simulink model "BMS"  (R2021a)
settings: Solver=FixedStepDiscrete  StartTime=0.0  StopTime=inf  FixedStep=1  RelTol=1e-3
values from neighbouring files (symbols this model uses):
  BattTempBp = [243.1 253.1 263.1 273.1 283.1 298.1 313.1]*0.1    [Variables.m]
  BM_TiCtctrCnct_P = single(1)/BMS_TiSample_C    [Variables.m]
  BM_TiCtctrDCnct_P = single(1)/BMS_TiSample_C    [Variables.m]
  BMS_EnaFltSts = [1 1 1 1 1 1 1 1 0 0 0 0 0]    [Variables.m]
  BMS_ModeEnaFltChk = [0 100 110 111 115 120 130 140 200 211 220 230 255]    [Variables.m]
  BMS_TiSample_C = single(0.1)    [Variables.m]
  BPC_BattTotalCharge_P = single(48)    [Variables.m]
  BPC_BattTotalEnergy_P = BPC_BattTotalCharge_P * single(NrCells_C) * CVM_VCellMaxCutoffTh_P    [Variables.m]
  CapLUTBp = [0 0.01 0.02 0.03 0.04 0.05 0.06 0.07 0.08 0.09 0.1 0.11 0.12 0.13 0.14 0.15 0.16 0.17 0.18 0.19 0.2 0.21 0.22 0.23 0.24 0.25 0.26 0.27 0.28 0.29 0.3 0.31 0.32 0.33 0.34 0.35 0.36 0.37 0.38 0.39 0.4 0.41 0.42 0.43 0.44 0.45 0.46 0.47 0.48 0.49 0.5 0.51 0.52 0.53 0.54 0.55 0.56 0.57 0.58 0.59 0.6 0.61 0.62 0.63 0.64 0.65 0.66 0.67 0.68 0.69 0.7 0.71 0.72 0.73 0.74 0.75 0.76 0.77 0.78 0.79 0.8 0.81  ...(+91 chars)    [Variables.m]
  CapSOCBp = [0 0.2 0.4 0.6 0.8 1]    [Variables.m]
  CVM_DMaxVCellMaxCutoff_P = int16(0.5/BMS_TiSample_C)    [Variables.m]
  CVM_DMaxVCellMaxDrtd_P = int16(0.5/BMS_TiSample_C)    [Variables.m]
  CVM_DMaxVCellMaxWarn_P = int16(0.5/BMS_TiSample_C)    [Variables.m]
  CVM_DMaxVCellMinCutoff_P = int16(0.5/BMS_TiSample_C)    [Variables.m]
  CVM_DMaxVCellMinDrtd_P = int16(0.5/BMS_TiSample_C)    [Variables.m]
  CVM_DMaxVCellMinWarn_P = int16(0.5/BMS_TiSample_C)    [Variables.m]
  CVM_DMinVCellMaxCutoff_P = -int16(0.5/BMS_TiSample_C)    [Variables.m]
  CVM_DMinVCellMaxDrtd_P = -int16(0.5/BMS_TiSample_C)    [Variables.m]
  CVM_DMinVCellMaxWarn_P = -int16(0.5/BMS_TiSample_C)    [Variables.m]
  CVM_DMinVCellMinCutoff_P = -int16(0.5/BMS_TiSample_C)    [Variables.m]
  CVM_DMinVCellMinDrtd_P = -int16(0.5/BMS_TiSample_C)    [Variables.m]
  CVM_DMinVCellMinWarn_P = -int16(0.5/BMS_TiSample_C)    [Variables.m]
  CVM_VCellMaxCutoffTh_P = single(4.22)    [Variables.m]
  CVM_VCellMaxDrtdTh_P = single(4.15)    [Variables.m]
  CVM_VCellMaxWarnTh_P = single(4.1)    [Variables.m]
  CVM_VCellMinCutoffTh_P = single(3.26)    [Variables.m]
  CVM_VCellMinDrtdTh_P = single(3)    [Variables.m]
  CVM_VCellMinWarnTh_P = single(2.8)    [Variables.m]
  Em = [2.8 3.228 3.284 3.361 3.408 3.427 3.472 3.477 3.493 3.504 3.516 3.528 3.537 3.545 3.555 3.561 3.566 3.576 3.587 3.589 3.594 3.6 3.608 3.61 3.616 3.619 3.626 3.632 3.637 3.64 3.645 3.646 3.652 3.655 3.658 3.661 3.664 3.668 3.673 3.678 3.68 3.681 3.686 3.692 3.699 3.702 3.705 3.71 3.717 3.723 3.728 3.733 3.735 3.742 3.749 3.755 3.761 3.768 3.773 3.78 3.791 3.798 3.798 3.814 3.818 3.825 3.841 3.846  ...(+196 chars)    [Variables.m]
  MTM_DMaxTMdulMaxCutoff_P = int16(0.5/BMS_TiSample_C)    [Variables.m]
  MTM_DMaxTMdulMaxDrtd_P = int16(0.5/BMS_TiSample_C)    [Variables.m]
  MTM_DMaxTMdulMaxWarn_P = int16(0.5/BMS_TiSample_C)    [Variables.m]
  MTM_DMaxTMdulMinCutoff_P = int16(0.5/BMS_TiSample_C)    [Variables.m]
  MTM_DMaxTMdulMinDrtd_P = int16(0.5/BMS_TiSample_C)    [Variables.m]
  MTM_DMaxTMdulMinWarn_P = int16(0.5/BMS_TiSample_C)    [Variables.m]
  MTM_DMinTMdulMaxCutoff_P = -int16(0.5/BMS_TiSample_C)    [Variables.m]
  MTM_DMinTMdulMaxDrtd_P = -int16(0.5/BMS_TiSample_C)    [Variables.m]
  MTM_DMinTMdulMaxWarn_P = -int16(0.5/BMS_TiSample_C)    [Variables.m]
  MTM_DMinTMdulMinCutoff_P = -int16(0.5/BMS_TiSample_C)    [Variables.m]
  MTM_DMinTMdulMinDrtd_P = -int16(0.5/BMS_TiSample_C)    [Variables.m]
  MTM_DMinTMdulMinWarn_P = -int16(0.5/BMS_TiSample_C)    [Variables.m]
  MTM_TMdulMaxCutoffTh_P = single(55)    [Variables.m]
  MTM_TMdulMaxDrtdTh_P = single(52.5)    [Variables.m]
  MTM_TMdulMaxWarnTh_P = single(50)    [Variables.m]
  MTM_TMdulMinCutoffTh_P = single(-20)    [Variables.m]
  MTM_TMdulMinDrtdTh_P = single(0)    [Variables.m]
  MTM_TMdulMinWarnTh_P = single(5)    [Variables.m]
  NrCutoff_C = uint8(3)    [Variables.m]
  NrDrtd_C = uint8(2)    [Variables.m]
  NrNoFlt_C = uint8(0)    [Variables.m]
  NrTMdulSnsr_C = uint8(3)    [Variables.m]
  NrWarn_C = uint8(1)    [Variables.m]
  RInt = [0.008846 0.009319 0.009027 0.00847 0.01032 0.01314;0.006389 0.006554 0.005553 0.005525 0.006043 0.007805;0.004364 0.004101 0.00406 0.003452 0.003846 0.004517;0.002031 0.002563 0.002532 0.00246 0.002716 0.003047;0.001443 0.001825 0.001795 0.001778 0.001924 0.002234;0.0005603 0.0007192 0.0006887 0.0007557 0.0007355 0.001014;0.001028 0.001338 0.001 0.001536 0.001546 0.002789]    [Variables.m]
undefined symbols (not defined in the file or in its folder): DiscIntNeverNeededParam
libraries: BMSLib x12
settings Model: Creator=Santosh  LastModifiedBy=Kuhan
settings SolverCC: AlgebraicLoopSolver=TrustRegion
settings DataIOCC: ReturnWorkspaceOutputs=off
settings DebuggingCC: SFMachineParentedDataDiag=warning  ArithmeticOperatorsInVariantConditions=warning
settings SFSimCC: CustomCodeUndefinedFunction=UseInterfaceOnly

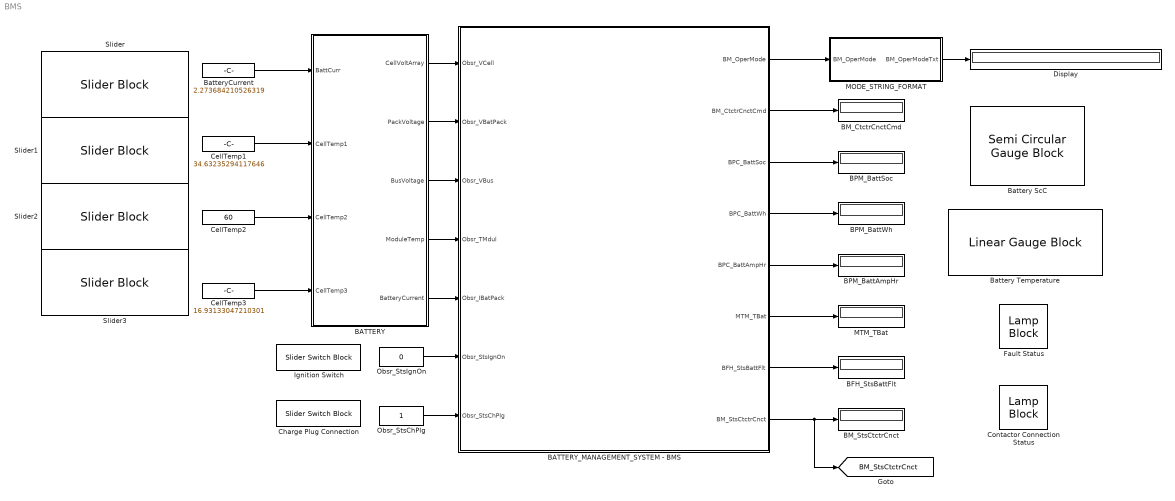
== system BMS ==
  BATTERY : Subsystem
  BATTERY_MANAGEMENT_SYSTEM - BMS : Subsystem
  BFH_StsBattFlt : Display
  BM_CtctrCnctCmd : Display
  BM_StsCtctrCnct : Display
  BPM_BattAmpHr : Display
  BPM_BattSoc : Display
  BPM_BattWh : Display
  Battery ScC : SemiCircularGaugeBlock
  Battery Temperature : LinearGaugeBlock  ScaleMin=-60  ScaleMax=60
  BatteryCurrent : Constant  Value=2.273684210526319  OutDataTypeStr=double
  CellTemp1 : Constant  Value=34.63235294117646  OutDataTypeStr=double
  CellTemp2 : Constant  Value=60  OutDataTypeStr=double
  CellTemp3 : Constant  Value=16.93133047210301  OutDataTypeStr=double
  Charge Plug Connection : SliderSwitchBlock
      settings: Values={{'Off', 'On'}, [0 1]}
  Contactor Connection Status : LampBlock
  Display : Display
  Fault Status : LampBlock
  Ignition Switch : SliderSwitchBlock
      settings: Values={{'Off', 'On'}, [0 1]}
  MODE_STRING_FORMAT : Subsystem
  MTM_TBat : Display
  Obsr_StsChPlg : Constant  OutDataTypeStr=boolean
  Obsr_StsIgnOn : Constant  Value=0  OutDataTypeStr=boolean
  Slider : SliderBlock  ScaleMin=-24  ScaleMax=24
  Slider1 : SliderBlock  ScaleMin=-30  ScaleMax=60
  Slider2 : SliderBlock  ScaleMin=-30  ScaleMax=60
  Slider3 : SliderBlock  ScaleMin=-30  ScaleMax=60
  tag scope: BM_StsCtctrCnct=global
  wires:
  Obsr_StsIgnOn/1 -> BATTERY_MANAGEMENT_SYSTEM - BMS/6(Obsr_StsIgnOn)
  Obsr_StsChPlg/1 -> BATTERY_MANAGEMENT_SYSTEM - BMS/7(Obsr_StsChPlg)
  BATTERY_MANAGEMENT_SYSTEM - BMS/3(BPC_BattSoc) -> BPM_BattSoc/1
  BATTERY_MANAGEMENT_SYSTEM - BMS/2(BM_CtctrCnctCmd) -> BM_CtctrCnctCmd/1
  BATTERY_MANAGEMENT_SYSTEM - BMS/4(BPC_BattWh) -> BPM_BattWh/1
  BATTERY_MANAGEMENT_SYSTEM - BMS/5(BPC_BattAmpHr) -> BPM_BattAmpHr/1
  BATTERY_MANAGEMENT_SYSTEM - BMS/6(MTM_TBat) -> MTM_TBat/1
  BATTERY_MANAGEMENT_SYSTEM - BMS/7(BFH_StsBattFlt) -> BFH_StsBattFlt/1
  BATTERY_MANAGEMENT_SYSTEM - BMS/8(BM_StsCtctrCnct) -> BM_StsCtctrCnct/1, [BM_StsCtctrCnct]
  BATTERY/1(CellVoltArray) -> BATTERY_MANAGEMENT_SYSTEM - BMS/1(Obsr_VCell)
  BATTERY/2(PackVoltage) -> BATTERY_MANAGEMENT_SYSTEM - BMS/2(Obsr_VBatPack)
  BATTERY/3(BusVoltage) -> BATTERY_MANAGEMENT_SYSTEM - BMS/3(Obsr_VBus)
  BATTERY/4(ModuleTemp) -> BATTERY_MANAGEMENT_SYSTEM - BMS/4(Obsr_TMdul)
  BATTERY/5(BatteryCurrent) -> BATTERY_MANAGEMENT_SYSTEM - BMS/5(Obsr_IBatPack)
  CellTemp1/1 -> BATTERY/2(CellTemp1)
  CellTemp2/1 -> BATTERY/3(CellTemp2)
  CellTemp3/1 -> BATTERY/4(CellTemp3)
  BATTERY_MANAGEMENT_SYSTEM - BMS/1(BM_OperMode) -> MODE_STRING_FORMAT/1(BM_OperMode)
  BatteryCurrent/1 -> BATTERY/1(BattCurr)
  MODE_STRING_FORMAT/1(BM_OperModeTxt) -> Display/1

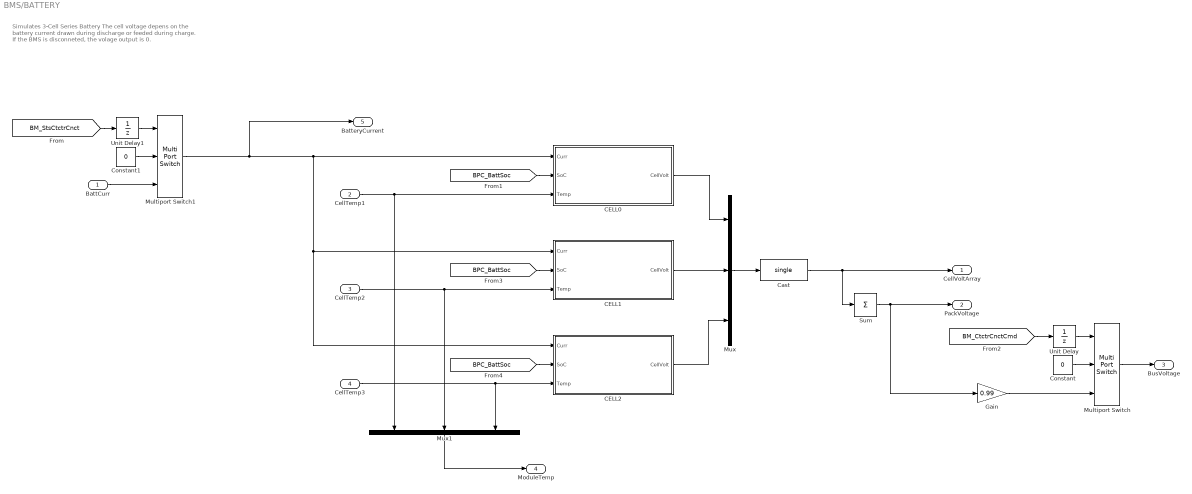
== system BMS/BATTERY ==
  note: Simulates 3-Cell Series Battery
      |
      | The cell voltage depens on the battery current drawn during discharge or feeded during charge.
      |
      | If the BMS is disconneted, the volage output is 0.
  BattCurr : Inport
  CellTemp1 : Inport  Port=2
  CellTemp2 : Inport  Port=3
  CellTemp3 : Inport  Port=4
  CELL0 : Subsystem
  CELL1 : Subsystem
  CELL2 : Subsystem
  Cast : DataTypeConversion  OutDataTypeStr=single
  Constant : Constant  Value=0
  Constant1 : Constant  Value=0
  Gain : Gain  Gain=0.99  OutDataTypeStr=single
  Multiport Switch : MultiPortSwitch  DataPortOrder=Zero-based contiguous  Inputs=2  zeroidx=on  OutDataTypeStr=single
  Multiport Switch1 : MultiPortSwitch  DataPortOrder=Zero-based contiguous  Inputs=2  zeroidx=on
  Mux : Mux  Inputs=3
  Mux1 : Mux  Inputs=3
  Sum : Sum  Inputs=1  AccumDataTypeStr=single
  Unit Delay : UnitDelay  SampleTime=-1  HasFrameUpgradeWarning=on
  Unit Delay1 : UnitDelay  SampleTime=-1  HasFrameUpgradeWarning=on
  CellVoltArray : Outport  VectorParamsAs1DForOutWhenUnconnected=off
  PackVoltage : Outport  Port=2  VectorParamsAs1DForOutWhenUnconnected=off
  BusVoltage : Outport  Port=3  VectorParamsAs1DForOutWhenUnconnected=off
  ModuleTemp : Outport  Port=4  VectorParamsAs1DForOutWhenUnconnected=off
  BatteryCurrent : Outport  Port=5  VectorParamsAs1DForOutWhenUnconnected=off
  wires:
  CellTemp2/1 -> CELL1/3(Temp), Mux1/2
  CELL1/1(CellVolt) -> Mux/2
  CellTemp3/1 -> CELL2/3(Temp), Mux1/3
  CELL2/1(CellVolt) -> Mux/3
  CELL0/1(CellVolt) -> Mux/1
  CellTemp1/1 -> CELL0/3(Temp), Mux1/1
  Mux/1 -> Cast/1
  Sum/1 -> PackVoltage/1, Gain/1
  Mux1/1 -> ModuleTemp/1
  Cast/1 -> Sum/1, CellVoltArray/1
  Multiport Switch1/1 -> CELL0/1(Curr), CELL2/1(Curr), CELL1/1(Curr), BatteryCurrent/1
  Unit Delay/1 -> Multiport Switch/1
  [BM_CtctrCnctCmd] -> Unit Delay/1
  Multiport Switch/1 -> BusVoltage/1
  Gain/1 -> Multiport Switch/3
  Constant/1 -> Multiport Switch/2
  Unit Delay1/1 -> Multiport Switch1/1
  [BM_StsCtctrCnct] -> Unit Delay1/1
  Constant1/1 -> Multiport Switch1/2
  BattCurr/1 -> Multiport Switch1/3
  [BPC_BattSoc] -> CELL0/2(SoC)
  [BPC_BattSoc] -> CELL1/2(SoC)
  [BPC_BattSoc] -> CELL2/2(SoC)

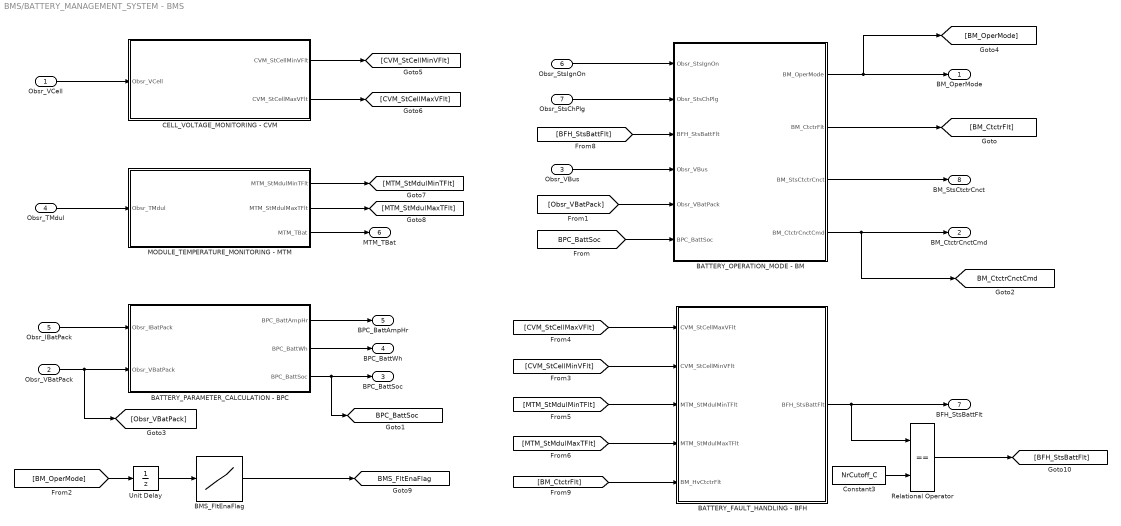
== system BMS/BATTERY_MANAGEMENT_SYSTEM - BMS ==
  Obsr_VCell : Inport
  Obsr_VBatPack : Inport  Port=2
  Obsr_VBus : Inport  Port=3
  Obsr_TMdul : Inport  Port=4
  Obsr_IBatPack : Inport  Port=5
  Obsr_StsIgnOn : Inport  Port=6
  Obsr_StsChPlg : Inport  Port=7
  BATTERY_FAULT_HANDLING - BFH : Subsystem
  BATTERY_OPERATION_MODE - BM : Subsystem
  BATTERY_PARAMETER_CALCULATION - BPC : Subsystem
  BMS_FltEnaFlag : Lookup_n-D  NumberOfTableDimensions=1  BreakpointsForDimension1=BMS_ModeEnaFltChk  Table=BMS_EnaFltSts  InterpMethod=Nearest  ExtrapMethod=Clip  DiagnosticForOutOfRangeInput=Error  InternalRulePriority=Speed  RndMeth=Simplest  InputSameDT=on
  CELL_VOLTAGE_MONITORING - CVM : Subsystem
  Constant3 : Constant  Value=NrCutoff_C
  MODULE_TEMPERATURE_MONITORING - MTM : Subsystem
  Relational Operator : RelationalOperator  Operator===  OutDataTypeStr=boolean  RndMeth=Simplest
  Unit Delay : UnitDelay  SampleTime=-1  HasFrameUpgradeWarning=on
  BM_OperMode : Outport  VectorParamsAs1DForOutWhenUnconnected=off
  BM_CtctrCnctCmd : Outport  Port=2  VectorParamsAs1DForOutWhenUnconnected=off
  BPC_BattSoc : Outport  Port=3  VectorParamsAs1DForOutWhenUnconnected=off
  BPC_BattWh : Outport  Port=4  VectorParamsAs1DForOutWhenUnconnected=off
  BPC_BattAmpHr : Outport  Port=5  VectorParamsAs1DForOutWhenUnconnected=off
  MTM_TBat : Outport  Port=6  VectorParamsAs1DForOutWhenUnconnected=off
  BFH_StsBattFlt : Outport  Port=7  VectorParamsAs1DForOutWhenUnconnected=off
  BM_StsCtctrCnct : Outport  Port=8  VectorParamsAs1DForOutWhenUnconnected=off
  tag scope: BMS_FltEnaFlag=global, BM_CtctrCnctCmd=global, BPC_BattSoc=global
  wires:
  Obsr_VCell/1 -> CELL_VOLTAGE_MONITORING - CVM/1(Obsr_VCell)
  Obsr_TMdul/1 -> MODULE_TEMPERATURE_MONITORING - MTM/1(Obsr_TMdul)
  [BPC_BattSoc] -> BATTERY_OPERATION_MODE - BM/6(BPC_BattSoc)
  Obsr_StsIgnOn/1 -> BATTERY_OPERATION_MODE - BM/1(Obsr_StsIgnOn)
  Obsr_StsChPlg/1 -> BATTERY_OPERATION_MODE - BM/2(Obsr_StsChPlg)
  [BFH_StsBattFlt] -> BATTERY_OPERATION_MODE - BM/3(BFH_StsBattFlt)
  Obsr_VBus/1 -> BATTERY_OPERATION_MODE - BM/4(Obsr_VBus)
  BATTERY_OPERATION_MODE - BM/4(BM_CtctrCnctCmd) -> BM_CtctrCnctCmd/1, [BM_CtctrCnctCmd]
  BATTERY_OPERATION_MODE - BM/2(BM_CtctrFlt) -> [BM_CtctrFlt]
  Obsr_VBatPack/1 -> [Obsr_VBatPack], BATTERY_PARAMETER_CALCULATION - BPC/2(Obsr_VBatPack)
  [Obsr_VBatPack] -> BATTERY_OPERATION_MODE - BM/5(Obsr_VBatPack)
  Obsr_IBatPack/1 -> BATTERY_PARAMETER_CALCULATION - BPC/1(Obsr_IBatPack)
  BATTERY_PARAMETER_CALCULATION - BPC/3(BPC_BattSoc) -> [BPC_BattSoc], BPC_BattSoc/1
  BATTERY_PARAMETER_CALCULATION - BPC/2(BPC_BattWh) -> BPC_BattWh/1
  BATTERY_PARAMETER_CALCULATION - BPC/1(BPC_BattAmpHr) -> BPC_BattAmpHr/1
  CELL_VOLTAGE_MONITORING - CVM/1(CVM_StCellMinVFlt) -> [CVM_StCellMinVFlt]
  CELL_VOLTAGE_MONITORING - CVM/2(CVM_StCellMaxVFlt) -> [CVM_StCellMaxVFlt]
  MODULE_TEMPERATURE_MONITORING - MTM/1(MTM_StMdulMinTFlt) -> [MTM_StMdulMinTFlt]
  MODULE_TEMPERATURE_MONITORING - MTM/2(MTM_StMdulMaxTFlt) -> [MTM_StMdulMaxTFlt]
  MODULE_TEMPERATURE_MONITORING - MTM/3(MTM_TBat) -> MTM_TBat/1
  [CVM_StCellMaxVFlt] -> BATTERY_FAULT_HANDLING - BFH/1(CVM_StCellMaxVFlt)
  [CVM_StCellMinVFlt] -> BATTERY_FAULT_HANDLING - BFH/2(CVM_StCellMinVFlt)
  [MTM_StMdulMinTFlt] -> BATTERY_FAULT_HANDLING - BFH/3(MTM_StMdulMinTFlt)
  [MTM_StMdulMaxTFlt] -> BATTERY_FAULT_HANDLING - BFH/4(MTM_StMdulMaxTFlt)
  BATTERY_FAULT_HANDLING - BFH/1(BFH_StsBattFlt) -> Relational Operator/1, BFH_StsBattFlt/1
  [BM_CtctrFlt] -> BATTERY_FAULT_HANDLING - BFH/5(BM_HvCtctrFlt)
  BATTERY_OPERATION_MODE - BM/3(BM_StsCtctrCnct) -> BM_StsCtctrCnct/1
  Relational Operator/1 -> [BFH_StsBattFlt]
  Constant3/1 -> Relational Operator/2
  BATTERY_OPERATION_MODE - BM/1(BM_OperMode) -> [BM_OperMode], BM_OperMode/1
  [BM_OperMode] -> Unit Delay/1
  BMS_FltEnaFlag/1 -> [BMS_FltEnaFlag]
  Unit Delay/1 -> BMS_FltEnaFlag/1

== system BMS/MODE_STRING_FORMAT ==
  BM_OperMode : Inport
  ASCII to String : ASCIIToString
  Cast : DataTypeConversion  OutDataTypeStr=uint8
  MATLAB Function : MATLAB Function  TreatAsAtomicUnit=on
  BM_OperModeTxt : Outport  VectorParamsAs1DForOutWhenUnconnected=off
  wires:
  Cast/1 -> ASCII to String/1
  ASCII to String/1 -> BM_OperModeTxt/1
  MATLAB Function/1(BmsModeText) -> Cast/1
  BM_OperMode/1 -> MATLAB Function/1(ModeNum)

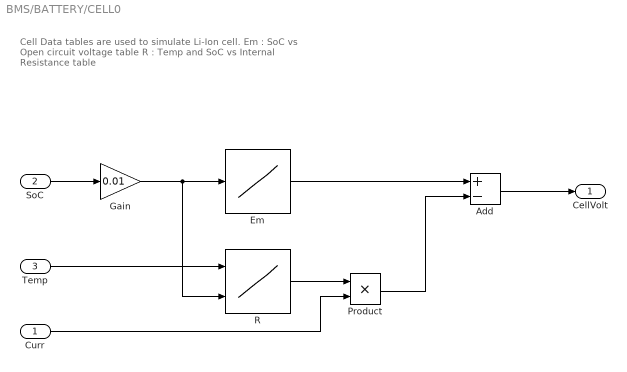
== system BMS/BATTERY/CELL0 ==
  note: Cell
      |
      | Data tables are used to simulate Li-Ion cell.
      |
      | Em : SoC vs Open circuit voltage table
      |
      | R : Temp and SoC vs Internal Resistance table
  Curr : Inport
  SoC : Inport  Port=2
  Temp : Inport  Port=3
  Add : Sum  Inputs=+-
  Em : Lookup_n-D  NumberOfTableDimensions=1  BreakpointsForDimension1=CapLUTBp  Table=Em  ExtrapMethod=Clip  UseLastTableValue=on  InternalRulePriority=Speed  RndMeth=Simplest  InputSameDT=on
  Gain : Gain  Gain=0.01  OutDataTypeStr=double
  Product : Product
  R : Lookup_n-D  BreakpointsForDimension1=BattTempBp  BreakpointsForDimension2=CapSOCBp  Table=RInt  ExtrapMethod=Clip  UseLastTableValue=on  InternalRulePriority=Speed  RndMeth=Simplest  InputSameDT=on
      settings: InputPortMap=u0,u1
  CellVolt : Outport  VectorParamsAs1DForOutWhenUnconnected=off
  wires:
  SoC/1 -> Gain/1
  Product/1 -> Add/2
  Curr/1 -> Product/2
  Add/1 -> CellVolt/1
  Temp/1 -> R/1
  R/1 -> Product/1
  Em/1 -> Add/1
  Gain/1 -> R/2, Em/1

== system BMS/BATTERY/CELL1 ==
  note: Cell
      |
      | Data tables are used to simulate Li-Ion cell.
      |
      | Em : SoC vs Open circuit voltage table
      |
      | R : Temp and SoC vs Internal Resistance table
  Curr : Inport
  SoC : Inport  Port=2
  Temp : Inport  Port=3
  Add : Sum  Inputs=+-
  Em : Lookup_n-D  NumberOfTableDimensions=1  BreakpointsForDimension1=CapLUTBp  Table=Em  InternalRulePriority=Speed  RndMeth=Simplest  InputSameDT=on
  Gain : Gain  Gain=0.01  OutDataTypeStr=double
  Product : Product
  R : Lookup_n-D  BreakpointsForDimension1=BattTempBp  BreakpointsForDimension2=CapSOCBp  Table=RInt  InternalRulePriority=Speed  RndMeth=Simplest  InputSameDT=on
      settings: InputPortMap=u0,u1
  CellVolt : Outport  VectorParamsAs1DForOutWhenUnconnected=off
  wires:
  Gain/1 -> Em/1, R/2
  Em/1 -> Add/1
  R/1 -> Product/1
  Temp/1 -> R/1
  Add/1 -> CellVolt/1
  Curr/1 -> Product/2
  Product/1 -> Add/2
  SoC/1 -> Gain/1

== system BMS/BATTERY/CELL2 ==
  note: Cell
      |
      | Data tables are used to simulate Li-Ion cell.
      |
      | Em : SoC vs Open circuit voltage table
      |
      | R : Temp and SoC vs Internal Resistance table
  Curr : Inport
  SoC : Inport  Port=2
  Temp : Inport  Port=3
  Add : Sum  Inputs=+-
  Em : Lookup_n-D  NumberOfTableDimensions=1  BreakpointsForDimension1=CapLUTBp  Table=Em  InternalRulePriority=Speed  RndMeth=Simplest  InputSameDT=on
  Gain : Gain  Gain=0.01  OutDataTypeStr=double
  Product : Product
  R : Lookup_n-D  BreakpointsForDimension1=BattTempBp  BreakpointsForDimension2=CapSOCBp  Table=RInt  InternalRulePriority=Speed  RndMeth=Simplest  InputSameDT=on
      settings: InputPortMap=u0,u1
  CellVolt : Outport  VectorParamsAs1DForOutWhenUnconnected=off
  wires:
  SoC/1 -> Gain/1
  Product/1 -> Add/2
  Curr/1 -> Product/2
  Add/1 -> CellVolt/1
  Temp/1 -> R/1
  R/1 -> Product/1
  Em/1 -> Add/1
  Gain/1 -> R/2, Em/1

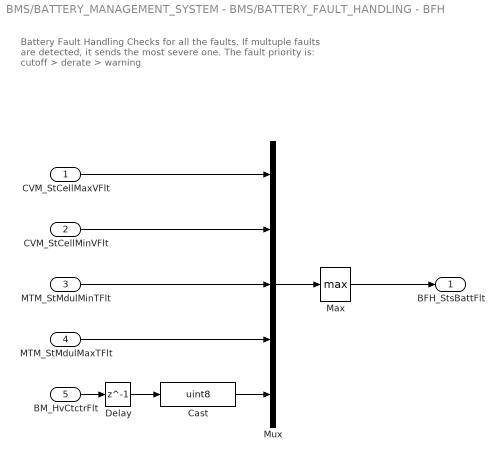
== system BMS/BATTERY_MANAGEMENT_SYSTEM - BMS/BATTERY_FAULT_HANDLING - BFH ==
  note: Battery Fault Handling
      |
      | Checks for all the faults. If multuple faults are detected, it sends the most severe one.
      |
      | The fault priority is: cutoff > derate > warning
  CVM_StCellMaxVFlt : Inport
  CVM_StCellMinVFlt : Inport  Port=2
  MTM_StMdulMinTFlt : Inport  Port=3
  MTM_StMdulMaxTFlt : Inport  Port=4
  BM_HvCtctrFlt : Inport  Port=5
  Cast : DataTypeConversion  OutDataTypeStr=uint8
  Delay : Delay  DelayLength=1
  Max : MinMax  Function=max  OutDataTypeStr=uint8
  Mux : Mux  Inputs=5
  BFH_StsBattFlt : Outport  VectorParamsAs1DForOutWhenUnconnected=off
  wires:
  Mux/1 -> Max/1
  MTM_StMdulMaxTFlt/1 -> Mux/4
  CVM_StCellMinVFlt/1 -> Mux/2
  CVM_StCellMaxVFlt/1 -> Mux/1
  MTM_StMdulMinTFlt/1 -> Mux/3
  Max/1 -> BFH_StsBattFlt/1
  BM_HvCtctrFlt/1 -> Delay/1
  Cast/1 -> Mux/5
  Delay/1 -> Cast/1

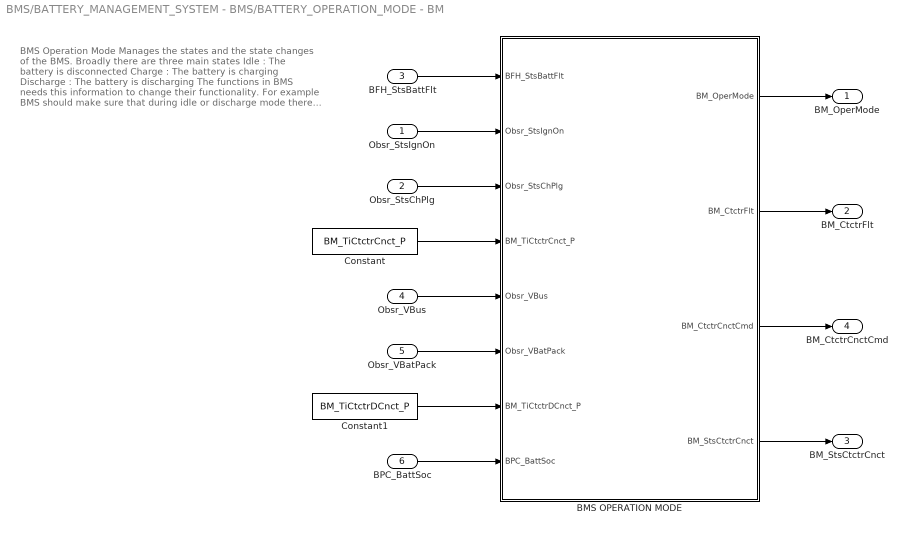
== system BMS/BATTERY_MANAGEMENT_SYSTEM - BMS/BATTERY_OPERATION_MODE - BM ==
  note: BMS Operation Mode
      |
      | Manages the states and the state changes of the BMS. Broadly there are three main states
      | Idle : The battery is disconnected
      | Charge : The battery is charging
      | Discharge : The battery is discharging
      |
      | The functions in BMS needs this information to change their functionality. For example BMS should make sure that during idle or discharge mode there is no current going into the battery. The SoC should increase during charge and decrease during discharge.
  Obsr_StsIgnOn : Inport
  Obsr_StsChPlg : Inport  Port=2
  BFH_StsBattFlt : Inport  Port=3
  Obsr_VBus : Inport  Port=4
  Obsr_VBatPack : Inport  Port=5
  BPC_BattSoc : Inport  Port=6
  BMS OPERATION MODE : Stateflow chart  TreatAsAtomicUnit=on
  Constant : Constant  Value=BM_TiCtctrCnct_P
  Constant1 : Constant  Value=BM_TiCtctrDCnct_P
  BM_OperMode : Outport  VectorParamsAs1DForOutWhenUnconnected=off
  BM_CtctrFlt : Outport  Port=2  VectorParamsAs1DForOutWhenUnconnected=off
  BM_StsCtctrCnct : Outport  Port=3  VectorParamsAs1DForOutWhenUnconnected=off
  BM_CtctrCnctCmd : Outport  Port=4  VectorParamsAs1DForOutWhenUnconnected=off
  wires:
  BFH_StsBattFlt/1 -> BMS OPERATION MODE/1(BFH_StsBattFlt)
  Obsr_StsIgnOn/1 -> BMS OPERATION MODE/2(Obsr_StsIgnOn)
  Obsr_StsChPlg/1 -> BMS OPERATION MODE/3(Obsr_StsChPlg)
  Obsr_VBus/1 -> BMS OPERATION MODE/5(Obsr_VBus)
  Obsr_VBatPack/1 -> BMS OPERATION MODE/6(Obsr_VBatPack)
  Constant/1 -> BMS OPERATION MODE/4(BM_TiCtctrCnct_P)
  Constant1/1 -> BMS OPERATION MODE/7(BM_TiCtctrDCnct_P)
  BMS OPERATION MODE/1(BM_OperMode) -> BM_OperMode/1
  BMS OPERATION MODE/2(BM_CtctrFlt) -> BM_CtctrFlt/1
  BMS OPERATION MODE/4(BM_StsCtctrCnct) -> BM_StsCtctrCnct/1
  BMS OPERATION MODE/3(BM_CtctrCnctCmd) -> BM_CtctrCnctCmd/1
  BPC_BattSoc/1 -> BMS OPERATION MODE/8(BPC_BattSoc)

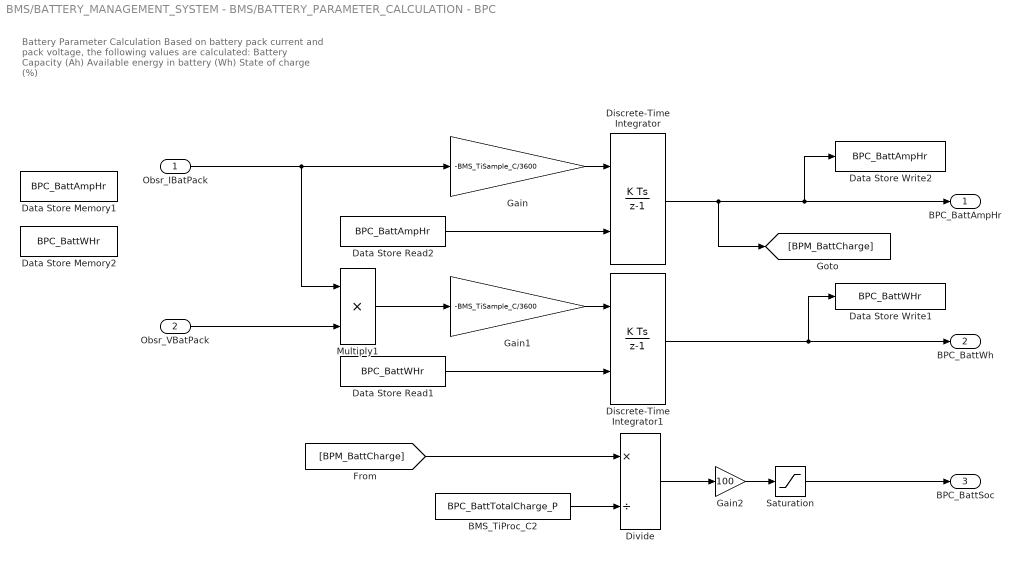
== system BMS/BATTERY_MANAGEMENT_SYSTEM - BMS/BATTERY_PARAMETER_CALCULATION - BPC ==
  note: Battery Parameter Calculation
      |
      | Based on battery pack current and pack voltage, the following values are calculated:
      | Battery Capacity (Ah)
      | Available energy in battery (Wh)
      | State of charge (%)
  Obsr_IBatPack : Inport
  Obsr_VBatPack : Inport  Port=2
  BMS_TiProc_C2 : Constant  Value=BPC_BattTotalCharge_P
  Data Store Memory1 : DataStoreMemory  DataStoreName=BPC_BattAmpHr  ReadBeforeWriteMsg=warning  WriteAfterWriteMsg=warning  WriteAfterReadMsg=warning  InitialValue=48*0.985  ShowAdditionalParam=off  OutDataTypeStr=double
  Data Store Memory2 : DataStoreMemory  DataStoreName=BPC_BattWHr  ReadBeforeWriteMsg=warning  WriteAfterWriteMsg=warning  WriteAfterReadMsg=warning  InitialValue=48*3*4.22*0.985  ShowAdditionalParam=off  OutDataTypeStr=double
  Data Store Read1 : DataStoreRead  DataStoreName=BPC_BattWHr  IndexOptions=Index vector (dialog)  Indices=1  OutputSizes=1
  Data Store Read2 : DataStoreRead  DataStoreName=BPC_BattAmpHr  IndexOptions=Index vector (dialog)  Indices=1  OutputSizes=1
  Data Store Write1 : DataStoreWrite  DataStoreName=BPC_BattWHr  IndexOptions=Index vector (dialog)  Indices=1  OutputSizes=1
  Data Store Write2 : DataStoreWrite  DataStoreName=BPC_BattAmpHr  IndexOptions=Index vector (dialog)  Indices=1  OutputSizes=1
  Discrete-Time Integrator : DiscreteIntegrator  InitialConditionSource=external  SampleTime=-1  LimitOutput=on  UpperSaturationLimit=BPC_BattTotalCharge_P  LowerSaturationLimit=0  ICPrevOutput=DiscIntNeverNeededParam  ICPrevScaledInput=DiscIntNeverNeededParam
  Discrete-Time Integrator1 : DiscreteIntegrator  InitialConditionSource=external  SampleTime=-1  LimitOutput=on  UpperSaturationLimit=BPC_BattTotalEnergy_P  LowerSaturationLimit=0  ICPrevOutput=DiscIntNeverNeededParam  ICPrevScaledInput=DiscIntNeverNeededParam
  Divide : Product  Inputs=*/  OutDataTypeStr=single
  Gain : Gain  Gain=-BMS_TiSample_C/3600  OutDataTypeStr=double
  Gain1 : Gain  Gain=-BMS_TiSample_C/3600  OutDataTypeStr=double
  Gain2 : Gain  Gain=100  OutMin=[0]  OutMax=[100]
  Multiply1 : Product
  Saturation : Saturate  UpperLimit=100  LowerLimit=0
  BPC_BattAmpHr : Outport  VectorParamsAs1DForOutWhenUnconnected=off
  BPC_BattWh : Outport  Port=2  VectorParamsAs1DForOutWhenUnconnected=off
  BPC_BattSoc : Outport  Port=3  VectorParamsAs1DForOutWhenUnconnected=off
  wires:
  Obsr_IBatPack/1 -> Multiply1/1, Gain/1
  Discrete-Time Integrator/1 -> [BPM_BattCharge], Data Store Write2/1, BPC_BattAmpHr/1
  Obsr_VBatPack/1 -> Multiply1/2
  Discrete-Time Integrator1/1 -> Data Store Write1/1, BPC_BattWh/1
  [BPM_BattCharge] -> Divide/1
  Divide/1 -> Gain2/1
  BMS_TiProc_C2/1 -> Divide/2
  Gain2/1 -> Saturation/1
  Saturation/1 -> BPC_BattSoc/1
  Multiply1/1 -> Gain1/1
  Data Store Read1/1 -> Discrete-Time Integrator1/2
  Data Store Read2/1 -> Discrete-Time Integrator/2
  Gain/1 -> Discrete-Time Integrator/1
  Gain1/1 -> Discrete-Time Integrator1/1

== system BMS/BATTERY_MANAGEMENT_SYSTEM - BMS/CELL_VOLTAGE_MONITORING - CVM ==
  note: Cell Voltage Monitoring
      |
      | Checks for cell over-voltage and under-voltage faults
  Obsr_VCell : Inport
  Max_Cell_Voltage_Fault_State : Subsystem
  Min : MinMax
  Min1 : MinMax  Function=max
  Min_Cell_Voltage_Fault_State : Subsystem
  CVM_StCellMinVFlt : Outport  VectorParamsAs1DForOutWhenUnconnected=off
  CVM_StCellMaxVFlt : Outport  Port=2  VectorParamsAs1DForOutWhenUnconnected=off
  wires:
  Obsr_VCell/1 -> Min/1, Min1/1
  Min/1 -> Min_Cell_Voltage_Fault_State/1(CVM_VCellMin)
  Min1/1 -> Max_Cell_Voltage_Fault_State/1(CVM_VCellMin)
  Min_Cell_Voltage_Fault_State/1(CVM_StCellMinVFlt) -> CVM_StCellMinVFlt/1
  Max_Cell_Voltage_Fault_State/1(CVM_StCellMaxVFlt) -> CVM_StCellMaxVFlt/1

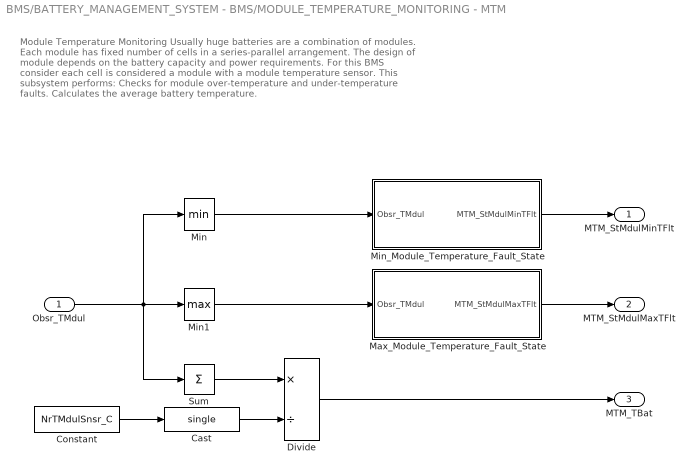
== system BMS/BATTERY_MANAGEMENT_SYSTEM - BMS/MODULE_TEMPERATURE_MONITORING - MTM ==
  note: Module Temperature Monitoring
      |
      | Usually huge batteries are a combination of modules. Each module has fixed number of cells in a series-parallel arrangement. The design of module depends on the battery capacity and power requirements. For this BMS consider each cell is considered a module with a module temperature sensor. This subsystem performs:
      |
      | Checks for module over-temperature and under-temperature faults.
      |
      | Calculates the average battery temperature.
  Obsr_TMdul : Inport
  Cast : DataTypeConversion  OutDataTypeStr=single
  Constant : Constant  Value=NrTMdulSnsr_C
  Divide : Product  Inputs=*/
  Max_Module_Temperature_Fault_State : Subsystem
  Min : MinMax
  Min1 : MinMax  Function=max
  Min_Module_Temperature_Fault_State : Subsystem
  Sum : Sum  Inputs=+
  MTM_StMdulMinTFlt : Outport  VectorParamsAs1DForOutWhenUnconnected=off
  MTM_StMdulMaxTFlt : Outport  Port=2  VectorParamsAs1DForOutWhenUnconnected=off
  MTM_TBat : Outport  Port=3  VectorParamsAs1DForOutWhenUnconnected=off
  wires:
  Min1/1 -> Max_Module_Temperature_Fault_State/1(Obsr_TMdul)
  Max_Module_Temperature_Fault_State/1(MTM_StMdulMaxTFlt) -> MTM_StMdulMaxTFlt/1
  Min/1 -> Min_Module_Temperature_Fault_State/1(Obsr_TMdul)
  Min_Module_Temperature_Fault_State/1(MTM_StMdulMinTFlt) -> MTM_StMdulMinTFlt/1
  Obsr_TMdul/1 -> Min/1, Sum/1, Min1/1
  Sum/1 -> Divide/1
  Divide/1 -> MTM_TBat/1
  Constant/1 -> Cast/1
  Cast/1 -> Divide/2

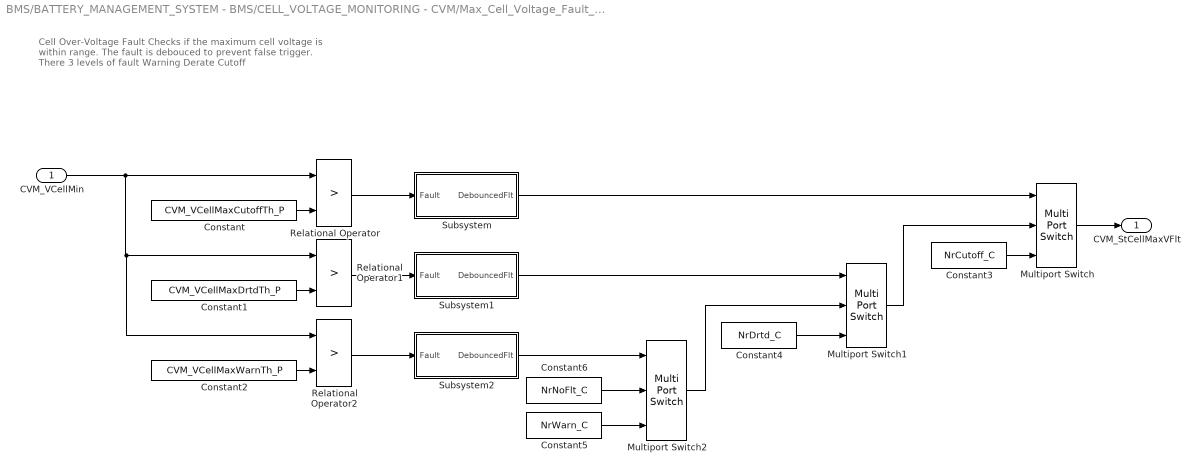
== system BMS/BATTERY_MANAGEMENT_SYSTEM - BMS/CELL_VOLTAGE_MONITORING - CVM/Max_Cell_Voltage_Fault_State ==
  note: Cell Over-Voltage Fault
      |
      | Checks if the maximum cell voltage is within range. The fault is debouced to prevent false trigger.
      |
      | There 3 levels of fault
      | Warning
      | Derate
      | Cutoff
  CVM_VCellMin : Inport
  Constant : Constant  Value=CVM_VCellMaxCutoffTh_P
  Constant1 : Constant  Value=CVM_VCellMaxDrtdTh_P
  Constant2 : Constant  Value=CVM_VCellMaxWarnTh_P
  Constant3 : Constant  Value=NrCutoff_C
  Constant4 : Constant  Value=NrDrtd_C
  Constant5 : Constant  Value=NrWarn_C
  Constant6 : Constant  Value=NrNoFlt_C
  Multiport Switch : MultiPortSwitch  DataPortOrder=Zero-based contiguous  Inputs=2  zeroidx=on
  Multiport Switch1 : MultiPortSwitch  DataPortOrder=Zero-based contiguous  Inputs=2  zeroidx=on
  Multiport Switch2 : MultiPortSwitch  DataPortOrder=Zero-based contiguous  Inputs=2  zeroidx=on
  Relational Operator : RelationalOperator  Operator=>  OutDataTypeStr=boolean  RndMeth=Simplest
  Relational Operator1 : RelationalOperator  Operator=>  OutDataTypeStr=boolean  RndMeth=Simplest
  Relational Operator2 : RelationalOperator  Operator=>  OutDataTypeStr=boolean  RndMeth=Simplest
  Subsystem : Subsystem
  Subsystem1 : Subsystem
  Subsystem2 : Subsystem
  CVM_StCellMaxVFlt : Outport  VectorParamsAs1DForOutWhenUnconnected=off
  wires:
  Constant6/1 -> Multiport Switch2/2
  Constant5/1 -> Multiport Switch2/3
  Constant2/1 -> Relational Operator2/2
  Multiport Switch2/1 -> Multiport Switch1/2
  Constant4/1 -> Multiport Switch1/3
  Constant1/1 -> Relational Operator1/2
  Constant3/1 -> Multiport Switch/3
  Multiport Switch1/1 -> Multiport Switch/2
  Constant/1 -> Relational Operator/2
  Multiport Switch/1 -> CVM_StCellMaxVFlt/1
  CVM_VCellMin/1 -> Relational Operator/1, Relational Operator1/1, Relational Operator2/1
  Relational Operator2/1 -> Subsystem2/1(Fault)
  Subsystem/1(DebouncedFlt) -> Multiport Switch/1
  Relational Operator/1 -> Subsystem/1(Fault)
  Relational Operator1/1 -> Subsystem1/1(Fault)
  Subsystem1/1(DebouncedFlt) -> Multiport Switch1/1
  Subsystem2/1(DebouncedFlt) -> Multiport Switch2/1

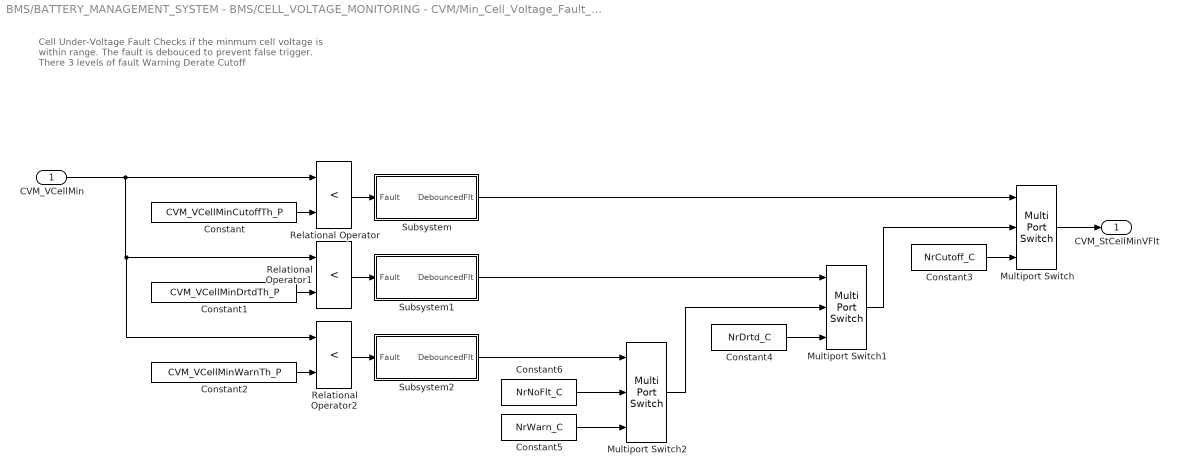
== system BMS/BATTERY_MANAGEMENT_SYSTEM - BMS/CELL_VOLTAGE_MONITORING - CVM/Min_Cell_Voltage_Fault_State ==
  note: Cell Under-Voltage Fault
      |
      | Checks if the minmum cell voltage is within range. The fault is debouced to prevent false trigger.
      |
      | There 3 levels of fault
      | Warning
      | Derate
      | Cutoff
  CVM_VCellMin : Inport
  Constant : Constant  Value=CVM_VCellMinCutoffTh_P
  Constant1 : Constant  Value=CVM_VCellMinDrtdTh_P
  Constant2 : Constant  Value=CVM_VCellMinWarnTh_P
  Constant3 : Constant  Value=NrCutoff_C
  Constant4 : Constant  Value=NrDrtd_C
  Constant5 : Constant  Value=NrWarn_C
  Constant6 : Constant  Value=NrNoFlt_C
  Multiport Switch : MultiPortSwitch  DataPortOrder=Zero-based contiguous  Inputs=2  zeroidx=on
  Multiport Switch1 : MultiPortSwitch  DataPortOrder=Zero-based contiguous  Inputs=2  zeroidx=on
  Multiport Switch2 : MultiPortSwitch  DataPortOrder=Zero-based contiguous  Inputs=2  zeroidx=on
  Relational Operator : RelationalOperator  Operator=<  OutDataTypeStr=boolean  RndMeth=Simplest
  Relational Operator1 : RelationalOperator  Operator=<  OutDataTypeStr=boolean  RndMeth=Simplest
  Relational Operator2 : RelationalOperator  Operator=<  OutDataTypeStr=boolean  RndMeth=Simplest
  Subsystem : Subsystem
  Subsystem1 : Subsystem
  Subsystem2 : Subsystem
  CVM_StCellMinVFlt : Outport  VectorParamsAs1DForOutWhenUnconnected=off
  wires:
  CVM_VCellMin/1 -> Relational Operator2/1, Relational Operator1/1, Relational Operator/1
  Multiport Switch/1 -> CVM_StCellMinVFlt/1
  Relational Operator/1 -> Subsystem/1(Fault)
  Constant/1 -> Relational Operator/2
  Multiport Switch1/1 -> Multiport Switch/2
  Constant3/1 -> Multiport Switch/3
  Relational Operator1/1 -> Subsystem1/1(Fault)
  Constant1/1 -> Relational Operator1/2
  Constant4/1 -> Multiport Switch1/3
  Multiport Switch2/1 -> Multiport Switch1/2
  Relational Operator2/1 -> Subsystem2/1(Fault)
  Constant2/1 -> Relational Operator2/2
  Constant5/1 -> Multiport Switch2/3
  Constant6/1 -> Multiport Switch2/2
  Subsystem/1(DebouncedFlt) -> Multiport Switch/1
  Subsystem1/1(DebouncedFlt) -> Multiport Switch1/1
  Subsystem2/1(DebouncedFlt) -> Multiport Switch2/1

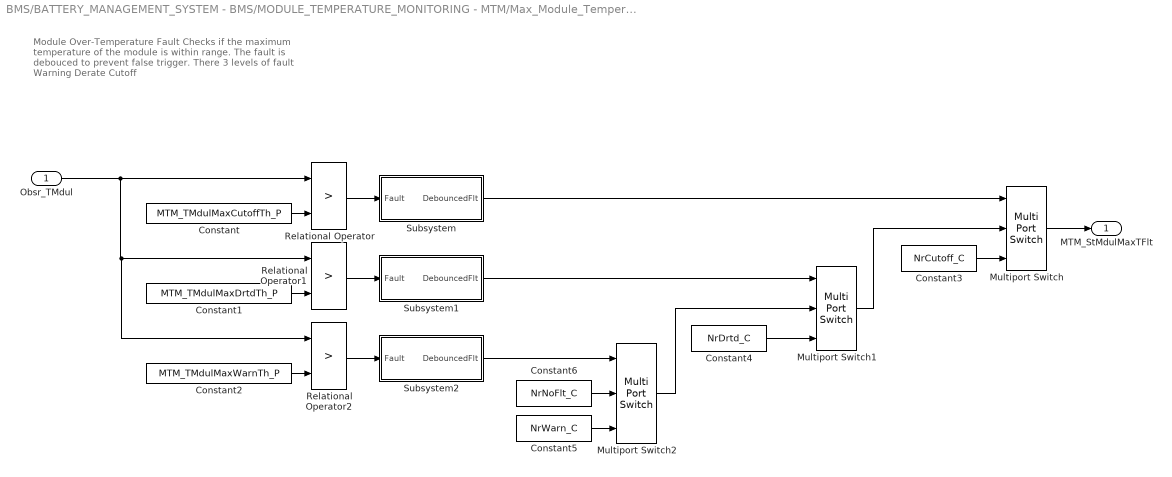
== system BMS/BATTERY_MANAGEMENT_SYSTEM - BMS/MODULE_TEMPERATURE_MONITORING - MTM/Max_Module_Temperature_Fault_State ==
  note: Module Over-Temperature Fault
      |
      | Checks if the maximum temperature of the module is within range. The fault is debouced to prevent false trigger.
      |
      | There 3 levels of fault
      | Warning
      | Derate
      | Cutoff
  Obsr_TMdul : Inport
  Constant : Constant  Value=MTM_TMdulMaxCutoffTh_P
  Constant1 : Constant  Value=MTM_TMdulMaxDrtdTh_P
  Constant2 : Constant  Value=MTM_TMdulMaxWarnTh_P
  Constant3 : Constant  Value=NrCutoff_C
  Constant4 : Constant  Value=NrDrtd_C
  Constant5 : Constant  Value=NrWarn_C
  Constant6 : Constant  Value=NrNoFlt_C
  Multiport Switch : MultiPortSwitch  DataPortOrder=Zero-based contiguous  Inputs=2  zeroidx=on
  Multiport Switch1 : MultiPortSwitch  DataPortOrder=Zero-based contiguous  Inputs=2  zeroidx=on
  Multiport Switch2 : MultiPortSwitch  DataPortOrder=Zero-based contiguous  Inputs=2  zeroidx=on
  Relational Operator : RelationalOperator  Operator=>  OutDataTypeStr=boolean  RndMeth=Simplest
  Relational Operator1 : RelationalOperator  Operator=>  OutDataTypeStr=boolean  RndMeth=Simplest
  Relational Operator2 : RelationalOperator  Operator=>  OutDataTypeStr=boolean  RndMeth=Simplest
  Subsystem : Subsystem
  Subsystem1 : Subsystem
  Subsystem2 : Subsystem
  MTM_StMdulMaxTFlt : Outport  VectorParamsAs1DForOutWhenUnconnected=off
  wires:
  Constant6/1 -> Multiport Switch2/2
  Constant5/1 -> Multiport Switch2/3
  Constant2/1 -> Relational Operator2/2
  Relational Operator2/1 -> Subsystem2/1(Fault)
  Multiport Switch2/1 -> Multiport Switch1/2
  Constant4/1 -> Multiport Switch1/3
  Constant1/1 -> Relational Operator1/2
  Relational Operator1/1 -> Subsystem1/1(Fault)
  Constant3/1 -> Multiport Switch/3
  Multiport Switch1/1 -> Multiport Switch/2
  Constant/1 -> Relational Operator/2
  Relational Operator/1 -> Subsystem/1(Fault)
  Multiport Switch/1 -> MTM_StMdulMaxTFlt/1
  Obsr_TMdul/1 -> Relational Operator/1, Relational Operator1/1, Relational Operator2/1
  Subsystem/1(DebouncedFlt) -> Multiport Switch/1
  Subsystem1/1(DebouncedFlt) -> Multiport Switch1/1
  Subsystem2/1(DebouncedFlt) -> Multiport Switch2/1

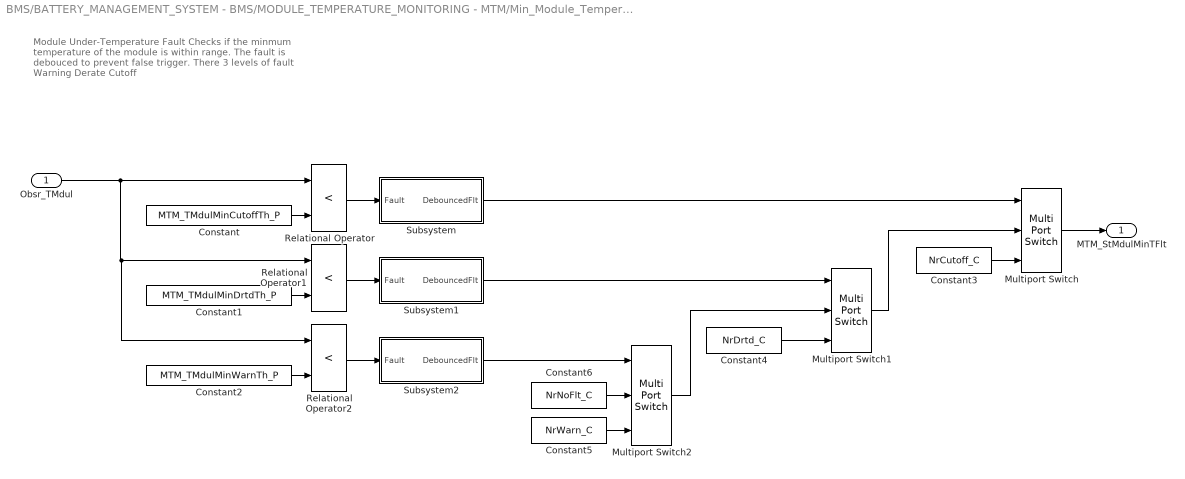
== system BMS/BATTERY_MANAGEMENT_SYSTEM - BMS/MODULE_TEMPERATURE_MONITORING - MTM/Min_Module_Temperature_Fault_State ==
  note: Module Under-Temperature Fault
      |
      | Checks if the minmum temperature of the module is within range. The fault is debouced to prevent false trigger.
      |
      | There 3 levels of fault
      | Warning
      | Derate
      | Cutoff
  Obsr_TMdul : Inport
  Constant : Constant  Value=MTM_TMdulMinCutoffTh_P
  Constant1 : Constant  Value=MTM_TMdulMinDrtdTh_P
  Constant2 : Constant  Value=MTM_TMdulMinWarnTh_P
  Constant3 : Constant  Value=NrCutoff_C
  Constant4 : Constant  Value=NrDrtd_C
  Constant5 : Constant  Value=NrWarn_C
  Constant6 : Constant  Value=NrNoFlt_C
  Multiport Switch : MultiPortSwitch  DataPortOrder=Zero-based contiguous  Inputs=2  zeroidx=on
  Multiport Switch1 : MultiPortSwitch  DataPortOrder=Zero-based contiguous  Inputs=2  zeroidx=on
  Multiport Switch2 : MultiPortSwitch  DataPortOrder=Zero-based contiguous  Inputs=2  zeroidx=on
  Relational Operator : RelationalOperator  Operator=<  OutDataTypeStr=boolean  RndMeth=Simplest
  Relational Operator1 : RelationalOperator  Operator=<  OutDataTypeStr=boolean  RndMeth=Simplest
  Relational Operator2 : RelationalOperator  Operator=<  OutDataTypeStr=boolean  RndMeth=Simplest
  Subsystem : Subsystem
  Subsystem1 : Subsystem
  Subsystem2 : Subsystem
  MTM_StMdulMinTFlt : Outport  VectorParamsAs1DForOutWhenUnconnected=off
  wires:
  Obsr_TMdul/1 -> Relational Operator2/1, Relational Operator1/1, Relational Operator/1
  Multiport Switch/1 -> MTM_StMdulMinTFlt/1
  Relational Operator/1 -> Subsystem/1(Fault)
  Constant/1 -> Relational Operator/2
  Multiport Switch1/1 -> Multiport Switch/2
  Constant3/1 -> Multiport Switch/3
  Relational Operator1/1 -> Subsystem1/1(Fault)
  Constant1/1 -> Relational Operator1/2
  Constant4/1 -> Multiport Switch1/3
  Multiport Switch2/1 -> Multiport Switch1/2
  Relational Operator2/1 -> Subsystem2/1(Fault)
  Constant2/1 -> Relational Operator2/2
  Constant5/1 -> Multiport Switch2/3
  Constant6/1 -> Multiport Switch2/2
  Subsystem/1(DebouncedFlt) -> Multiport Switch/1
  Subsystem1/1(DebouncedFlt) -> Multiport Switch1/1
  Subsystem2/1(DebouncedFlt) -> Multiport Switch2/1

== system BMS/BATTERY_MANAGEMENT_SYSTEM - BMS/CELL_VOLTAGE_MONITORING - CVM/Max_Cell_Voltage_Fault_State/Subsystem ==
  Fault : Inport
  Constant : Constant  Value=0
  Constant2 : Constant  Value=CVM_DMaxVCellMaxCutoff_P
  Constant3 : Constant  Value=CVM_DMinVCellMaxCutoff_P
  Subsystem : BMSLib/Debouncer
  DebouncedFlt : Outport  VectorParamsAs1DForOutWhenUnconnected=off
  wires:
  Fault/1 -> Subsystem/1
  Subsystem/1 -> DebouncedFlt/1
  [BMS_FltEnaFlag] -> Subsystem/2
  Constant/1 -> Subsystem/3
  Constant2/1 -> Subsystem/4
  Constant3/1 -> Subsystem/5

== system BMS/BATTERY_MANAGEMENT_SYSTEM - BMS/CELL_VOLTAGE_MONITORING - CVM/Max_Cell_Voltage_Fault_State/Subsystem1 ==
  Fault : Inport
  Constant1 : Constant  Value=0
  Constant2 : Constant  Value=CVM_DMaxVCellMaxDrtd_P
  Constant3 : Constant  Value=CVM_DMinVCellMaxDrtd_P
  Subsystem : BMSLib/Debouncer
  DebouncedFlt : Outport  VectorParamsAs1DForOutWhenUnconnected=off
  wires:
  Constant3/1 -> Subsystem/5
  Constant2/1 -> Subsystem/4
  Constant1/1 -> Subsystem/3
  [BMS_FltEnaFlag] -> Subsystem/2
  Subsystem/1 -> DebouncedFlt/1
  Fault/1 -> Subsystem/1

== system BMS/BATTERY_MANAGEMENT_SYSTEM - BMS/CELL_VOLTAGE_MONITORING - CVM/Max_Cell_Voltage_Fault_State/Subsystem2 ==
  Fault : Inport
  Constant1 : Constant  Value=0
  Constant2 : Constant  Value=CVM_DMaxVCellMaxWarn_P
  Constant3 : Constant  Value=CVM_DMinVCellMaxWarn_P
  Subsystem : BMSLib/Debouncer
  DebouncedFlt : Outport  VectorParamsAs1DForOutWhenUnconnected=off
  wires:
  Fault/1 -> Subsystem/1
  Subsystem/1 -> DebouncedFlt/1
  [BMS_FltEnaFlag] -> Subsystem/2
  Constant1/1 -> Subsystem/3
  Constant2/1 -> Subsystem/4
  Constant3/1 -> Subsystem/5

== system BMS/BATTERY_MANAGEMENT_SYSTEM - BMS/CELL_VOLTAGE_MONITORING - CVM/Min_Cell_Voltage_Fault_State/Subsystem ==
  Fault : Inport
  Constant1 : Constant  Value=0
  Constant2 : Constant  Value=CVM_DMaxVCellMinCutoff_P
  Constant3 : Constant  Value=CVM_DMinVCellMinCutoff_P
  Subsystem : BMSLib/Debouncer
  DebouncedFlt : Outport  VectorParamsAs1DForOutWhenUnconnected=off
  wires:
  Fault/1 -> Subsystem/1
  Subsystem/1 -> DebouncedFlt/1
  [BMS_FltEnaFlag] -> Subsystem/2
  Constant1/1 -> Subsystem/3
  Constant2/1 -> Subsystem/4
  Constant3/1 -> Subsystem/5

== system BMS/BATTERY_MANAGEMENT_SYSTEM - BMS/CELL_VOLTAGE_MONITORING - CVM/Min_Cell_Voltage_Fault_State/Subsystem1 ==
  Fault : Inport
  Constant1 : Constant  Value=0
  Constant2 : Constant  Value=CVM_DMaxVCellMinDrtd_P
  Constant3 : Constant  Value=CVM_DMinVCellMinDrtd_P
  Subsystem : BMSLib/Debouncer
  DebouncedFlt : Outport  VectorParamsAs1DForOutWhenUnconnected=off
  wires:
  Constant3/1 -> Subsystem/5
  Constant2/1 -> Subsystem/4
  Constant1/1 -> Subsystem/3
  [BMS_FltEnaFlag] -> Subsystem/2
  Subsystem/1 -> DebouncedFlt/1
  Fault/1 -> Subsystem/1

== system BMS/BATTERY_MANAGEMENT_SYSTEM - BMS/CELL_VOLTAGE_MONITORING - CVM/Min_Cell_Voltage_Fault_State/Subsystem2 ==
  Fault : Inport
  Constant1 : Constant  Value=0
  Constant2 : Constant  Value=CVM_DMaxVCellMinWarn_P
  Constant3 : Constant  Value=CVM_DMinVCellMinWarn_P
  Subsystem : BMSLib/Debouncer
  DebouncedFlt : Outport  VectorParamsAs1DForOutWhenUnconnected=off
  wires:
  Fault/1 -> Subsystem/1
  Subsystem/1 -> DebouncedFlt/1
  [BMS_FltEnaFlag] -> Subsystem/2
  Constant1/1 -> Subsystem/3
  Constant2/1 -> Subsystem/4
  Constant3/1 -> Subsystem/5

== system BMS/BATTERY_MANAGEMENT_SYSTEM - BMS/MODULE_TEMPERATURE_MONITORING - MTM/Max_Module_Temperature_Fault_State/Subsystem ==
  Fault : Inport
  Constant1 : Constant  Value=0
  Constant2 : Constant  Value=MTM_DMaxTMdulMaxCutoff_P
  Constant3 : Constant  Value=MTM_DMinTMdulMaxCutoff_P
  Subsystem : BMSLib/Debouncer
  DebouncedFlt : Outport  VectorParamsAs1DForOutWhenUnconnected=off
  wires:
  Fault/1 -> Subsystem/1
  Subsystem/1 -> DebouncedFlt/1
  [BMS_FltEnaFlag] -> Subsystem/2
  Constant1/1 -> Subsystem/3
  Constant2/1 -> Subsystem/4
  Constant3/1 -> Subsystem/5

== system BMS/BATTERY_MANAGEMENT_SYSTEM - BMS/MODULE_TEMPERATURE_MONITORING - MTM/Max_Module_Temperature_Fault_State/Subsystem1 ==
  Fault : Inport
  Constant1 : Constant  Value=0
  Constant2 : Constant  Value=MTM_DMaxTMdulMaxDrtd_P
  Constant3 : Constant  Value=MTM_DMinTMdulMaxDrtd_P
  Subsystem : BMSLib/Debouncer
  DebouncedFlt : Outport  VectorParamsAs1DForOutWhenUnconnected=off
  wires:
  Constant3/1 -> Subsystem/5
  Constant2/1 -> Subsystem/4
  Constant1/1 -> Subsystem/3
  [BMS_FltEnaFlag] -> Subsystem/2
  Subsystem/1 -> DebouncedFlt/1
  Fault/1 -> Subsystem/1

== system BMS/BATTERY_MANAGEMENT_SYSTEM - BMS/MODULE_TEMPERATURE_MONITORING - MTM/Max_Module_Temperature_Fault_State/Subsystem2 ==
  Fault : Inport
  Constant1 : Constant  Value=0
  Constant2 : Constant  Value=MTM_DMaxTMdulMaxWarn_P
  Constant3 : Constant  Value=MTM_DMinTMdulMaxWarn_P
  Subsystem : BMSLib/Debouncer
  DebouncedFlt : Outport  VectorParamsAs1DForOutWhenUnconnected=off
  wires:
  Fault/1 -> Subsystem/1
  Subsystem/1 -> DebouncedFlt/1
  [BMS_FltEnaFlag] -> Subsystem/2
  Constant1/1 -> Subsystem/3
  Constant2/1 -> Subsystem/4
  Constant3/1 -> Subsystem/5

== system BMS/BATTERY_MANAGEMENT_SYSTEM - BMS/MODULE_TEMPERATURE_MONITORING - MTM/Min_Module_Temperature_Fault_State/Subsystem ==
  Fault : Inport
  Constant1 : Constant  Value=0
  Constant2 : Constant  Value=MTM_DMaxTMdulMinCutoff_P
  Constant3 : Constant  Value=MTM_DMinTMdulMinCutoff_P
  Subsystem : BMSLib/Debouncer
  DebouncedFlt : Outport  VectorParamsAs1DForOutWhenUnconnected=off
  wires:
  Fault/1 -> Subsystem/1
  Subsystem/1 -> DebouncedFlt/1
  [BMS_FltEnaFlag] -> Subsystem/2
  Constant1/1 -> Subsystem/3
  Constant2/1 -> Subsystem/4
  Constant3/1 -> Subsystem/5

== system BMS/BATTERY_MANAGEMENT_SYSTEM - BMS/MODULE_TEMPERATURE_MONITORING - MTM/Min_Module_Temperature_Fault_State/Subsystem1 ==
  Fault : Inport
  Constant1 : Constant  Value=0
  Constant2 : Constant  Value=MTM_DMaxTMdulMinDrtd_P
  Constant3 : Constant  Value=MTM_DMinTMdulMinDrtd_P
  Subsystem : BMSLib/Debouncer
  DebouncedFlt : Outport  VectorParamsAs1DForOutWhenUnconnected=off
  wires:
  Constant3/1 -> Subsystem/5
  Constant2/1 -> Subsystem/4
  Constant1/1 -> Subsystem/3
  [BMS_FltEnaFlag] -> Subsystem/2
  Subsystem/1 -> DebouncedFlt/1
  Fault/1 -> Subsystem/1

== system BMS/BATTERY_MANAGEMENT_SYSTEM - BMS/MODULE_TEMPERATURE_MONITORING - MTM/Min_Module_Temperature_Fault_State/Subsystem2 ==
  Fault : Inport
  Constant1 : Constant  Value=0
  Constant2 : Constant  Value=MTM_DMaxTMdulMinWarn_P
  Constant3 : Constant  Value=MTM_DMinTMdulMinWarn_P
  Subsystem : BMSLib/Debouncer
  DebouncedFlt : Outport  VectorParamsAs1DForOutWhenUnconnected=off
  wires:
  Fault/1 -> Subsystem/1
  Subsystem/1 -> DebouncedFlt/1
  [BMS_FltEnaFlag] -> Subsystem/2
  Constant1/1 -> Subsystem/3
  Constant2/1 -> Subsystem/4
  Constant3/1 -> Subsystem/5

== matlab function BMS/MODE_STRING_FORMAT/MATLAB Function ==
  data: ModeNum input; BmsModeText output
function BmsModeText = BmsMode(ModeNum)
    if(ModeNum == 100)
        BmsModeText = [73 100 108 101 zeros(1,24)];
    elseif(ModeNum == 110)
        BmsModeText = [67 111 110 116 97 99 116 111 114 32 67 111 110 110 101 99 116 32 67 111 109 109 97 110 100 zeros(1,3)];
    elseif(ModeNum == 111)
        BmsModeText = [67 111 110 116 97 99 116 111 114 32 67 111 110 110 101 99 116 32 67 104 101 99 107 zeros(1,5)];
    elseif(ModeNum == 115)
        BmsModeText = [67 111 110 116 97 99 116 111 114 32 67 111 110 110 101 99 116 32 70 97 105 108 zeros(1,6)];
    elseif(ModeNum == 120)
        BmsModeText = [67 111 110 116 97 99 116 111 114 32 67 111 110 110 101 99 116 101 100 zeros(1,9)];
    elseif(ModeNum == 130)
        BmsModeText = [67 104 97 114 103 105 110 103 zeros(1,20)];
    elseif(ModeNum == 140)
        BmsModeText = [68 105 115 99 104 97 114 103 105 110 103 zeros(1,17)];
    elseif(ModeNum == 200)
        BmsModeText = [67 111 110 116 97 99 116 111 114 32 68 105 115 99 111 110 110 101 99 116 32 67 111 109 109 97 110 100];
    elseif(ModeNum == 211)
        BmsModeText = [67 111 110 116 97 99 116 111 114 32 68 105 115 99 111 110 110 101 99 116 32 67 104 101 99 107 zeros(1,2)];
    elseif(ModeNum == 230)
        BmsModeText = [67 111 110 116 97 99 116 111 114 32 68 105 115 99 111 110 110 101 99 116 32 70 97 105 108 zeros(1,3)];
    elseif(ModeNum == 240)
        BmsModeText = [67 111 110 116 97 99 116 111 114 32 68 105 115 99 111 110 110 101 99 116 32 83 117 99 99 101 115 115];
    else
        BmsModeText = [73 100 108 101 zeros(1,24)];
    end
end

== stateflow chart BMS/BATTERY_MANAGEMENT_SYSTEM - BMS/BATTERY_OPERATION_MODE - BM/BMS OPERATION MODE ==
  state IDLE
    entry:
    BM_OperMode = 100;
    BM_CtctrCnctCmd = false;
  state CONTACTOR_CONNECT_COMMAND
    entry:
    BM_OperMode = 110;
    BM_CtctrCnctCmd = true;
  state FAULT
    entry:
    BM_OperMode = 255;
    BM_CtctrCnctCmd = false;
  state CONTACTOR_CONNECT_FAIL
    entry:
    BM_OperMode = 115;
    BM_CtctrFlt = true;
  state CONTACTOR_CONNECT_CHECK
    entry:
    BM_OperMode = 111;
  state CONTACTOR_CONNECT_SEQUENCE
    state CONTACTOR_CONNECT_SUCCESS
      entry:
      BM_OperMode = 120;
      BM_StsCtctrCnct = true;
    state CHARGING
      entry:
      BM_OperMode = 130;
    state DISCHARGING
      entry:
      BM_OperMode = 140;
    CONTACTOR_CONNECT_SUCCESS -> CHARGING [order 1] : [Obsr_StsChPlg == true]
    CONTACTOR_CONNECT_SUCCESS -> DISCHARGING [order 2] : [Obsr_StsIgnOn == true]
    DISCHARGING -> CHARGING [order 1] : [Obsr_StsChPlg == true]
    CHARGING -> DISCHARGING [order 1] : [(Obsr_StsChPlg == false) && (Obsr_StsIgnOn == true)]
  state CONTACTOR_DICCONNECT_CHECK
    entry:
    BM_OperMode = 211;
  state CONTACTOR_DISCONNECT_FAIL
    entry:
    BM_OperMode = 230;
    BM_CtctrFlt = true;
  state CONTACTOR_DISCONNECT_COMMAND
    entry:
    BM_OperMode = 200;
    BM_CtctrCnctCmd = false;
  state CONTACTOR_DISCONNECT_SUCCESS
    entry:
    BM_OperMode = 220;
    BM_StsCtctrCnct = false;
  DISCHARGING -> CONTACTOR_DISCONNECT_COMMAND [order 2] : [((Obsr_StsIgnOn == false)||(BPC_BattSoc < 3 ))]
  CHARGING -> CONTACTOR_DISCONNECT_COMMAND [order 2] : [(Obsr_StsChPlg == false)||(BPC_BattSoc >= 98.5 )]
  (default) -> IDLE : {BM_CtctrFlt = false;
      | BM_StsCtctrCnct = false;}
  IDLE -> (junction 41) : [BFH_StsBattFlt == false]
  (junction 80) -> IDLE
  (junction 41) -> CONTACTOR_CONNECT_COMMAND : [((Obsr_StsIgnOn == true)&&(BPC_BattSoc > 3 ))||((Obsr_StsChPlg == true)&&(BPC_BattSoc < 98.5))]
  (junction 77) -> (junction 80)
  CONTACTOR_CONNECT_COMMAND -> CONTACTOR_CONNECT_CHECK : [after(BM_TiCtctrCnct_P,tick)]
  FAULT -> (junction 77) : [(Obsr_StsIgnOn == false) && (Obsr_StsChPlg == false)]
  (junction 96) -> (junction 77)
  CONTACTOR_CONNECT_FAIL -> FAULT
  CONTACTOR_CONNECT_CHECK -> CONTACTOR_CONNECT_FAIL [order 1] : [Obsr_VBus < 0.98*Obsr_VBatPack]
  CONTACTOR_DISCONNECT_FAIL -> FAULT
  CONTACTOR_DISCONNECT_SUCCESS -> FAULT [order 1] : [BFH_StsBattFlt == true]
  CONTACTOR_CONNECT_CHECK -> CONTACTOR_CONNECT_SUCCESS [order 2] : [Obsr_VBus >= 0.95*Obsr_VBatPack]
  CONTACTOR_CONNECT_SEQUENCE -> CONTACTOR_DISCONNECT_COMMAND : [BFH_StsBattFlt == true]
  CONTACTOR_DICCONNECT_CHECK -> CONTACTOR_DISCONNECT_FAIL [order 2]
  CONTACTOR_DISCONNECT_COMMAND -> CONTACTOR_DICCONNECT_CHECK : [after(BM_TiCtctrDCnct_P,tick)]
  CONTACTOR_DICCONNECT_CHECK -> CONTACTOR_DISCONNECT_SUCCESS [order 1] : [Obsr_VBus < 0.2*Obsr_VBatPack]
  CONTACTOR_DISCONNECT_SUCCESS -> (junction 96) [order 2]
  data: BFH_StsBattFlt input boolean; Obsr_StsIgnOn input boolean; Obsr_StsChPlg input boolean; BM_TiCtctrCnct_P input single; Obsr_VBus input single; Obsr_VBatPack input single; BM_TiCtctrDCnct_P input single; BM_OperMode output uint8; BM_CtctrFlt output boolean; BM_CtctrCnctCmd output boolean; BM_StsCtctrCnct output boolean; BPC_BattSoc input single
